simulink model "MotorControlLibSim"  (R2020b)
settings: Solver=FixedStepDiscrete  StartTime=0.0  StopTime=10  FixedStep=1e-6  RelTol=1e-3
undefined symbols (not defined in the file): BrkPoints, d_q_Voltage_Limiter_max, DiscIntNeverNeededParam, Down, dSoll, Ki_dAxis, Ki_qAxis, Kp_dAxis, Kp_qAxis, NumBits1, NumBits2, polepairs, pwmTableData, qSoll, Slope1, Slope2, TqToIqConst, Ts, Up
libraries: simulink x6, eePwmGenerator x3, simulink_extras x2, autolibpmsminterior x1
settings Model: DataDictionary=MotorControl.sldd  NumberOfSteps=10  Creator=unix  LastModifiedBy=unix
settings SolverCC: AutoInsertRateTranBlk=on
settings OptimizationCC: DefaultParameterBehavior=Inlined  EnhancedBackFolding=on  PassReuseOutputArgsAs=Individual arguments  ZeroExternalMemoryAtStartup=off  ZeroInternalMemoryAtStartup=off  OptimizeBlockOrder=speed  DifferentSizesBufferReuse=on  OptimizationCustomize=off  EfficientTunableParamExpr=on
settings DebuggingCC: ArrayBoundsChecking=warning  SignalInfNanChecking=warning  SignalRangeChecking=warning  CheckMatrixSingularityMsg=warning  IntegerOverflowMsg=error  ParameterOverflowMsg=warning  ParameterUnderflowMsg=warning  ParameterPrecisionLossMsg=none  ParameterTunabilityLossMsg=error  UnderSpecifiedDataTypeMsg=warning  IntegerSaturationMsg=error
settings SFSimCC: MATLABDynamicMemAlloc=off
settings RTWCC: Description=Embedded Coder  SystemTargetFile=ert.tlc  GenCodeOnly=on  TemplateMakefile=ert_default_tmf  GenerateReport=on  IncludeHyperlinkInReport=on  LaunchReport=on  GenerateTraceInfo=on  GenerateTraceReport=on  GenerateTraceReportSl=on  GenerateTraceReportSf=on  GenerateTraceReportEml=on
settings CodeAppCC: ForceParamTrailComments=on  IgnoreCustomStorageClasses=off  OperatorAnnotations=on  SimulinkDataObjDesc=on  SFDataObjDesc=on  InsertBlockDesc=on
settings ERTTargetCC: TargetLangStandard=C99 (ISO)  GenerateSampleERTMain=on  GenerateASAP2=on  InlinedParameterPlacement=NonHierarchical  ERTCustomFileTemplate=example_file_process.tlc

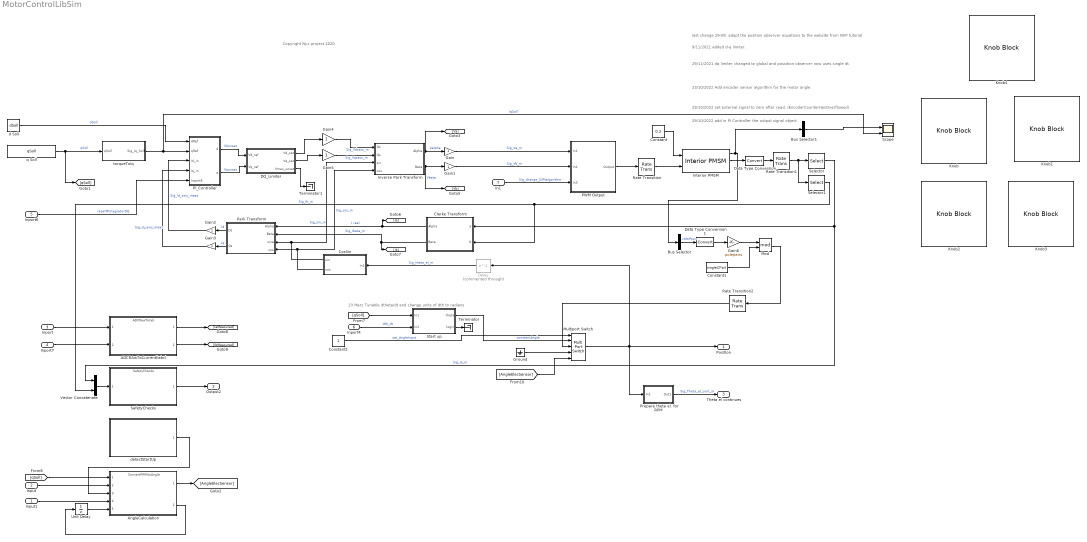
== system MotorControlLibSim ==
  note: Copyright Nyx project 2020
  note: 29/11/2021 dq limiter changed to global and possition observer now uses single dt.
  note: 9/11/2021 added d-q limiter.
  note: last change 29-08: adapt the position observer equations to the website from NXP tutorial
  note: 23 Marz Tunable dtheta/dt and change units of dth to radians
  note: 23/10/2022 Add encoder sensor algorithm for the motor angle
  note: 29/10/2022 set external signal to zero after read, (EncoderCounterHasOverflowed)
  note: 29/10/2022 add in PI Controller the output signal object
  Input1 : Inport
  Input : Inport  Port=2
  Inport : Inport  Port=3
  Inport7 : Inport  Port=4
  Inport6 : Inport  Port=5  OutDataTypeStr=boolean
  Inport4 : Inport  Port=6
  In1 : Inport  Port=7
  ADCRAwToCurrent(Iabc) : ModelReference  ModelNameDialog=ADCRawToIab  ModelReferenceVersion=3.11
  AngleCalculation : ModelReference  ModelNameDialog=ConvertPWMtoAngle.slx  ModelReferenceVersion=3.7
  Bus Selector : BusSelector  OutputSignals=MtrPos
  Bus Selector1 : BusSelector  OutputSignals=MtrPos,IcStator,IbStator,IaStator  OutputAsBus=on
  Clarke Transform : Subsystem  VariantControl=Variant2  mask(Clarke Transform){}
      mask help:
      | <p>Compute Clarke transformation on balanced 3-phase inputs into balanced 2-phase orthogonal outputs.
      | <br>
      | <br>
      | The block accepts two signals out of three phases, and outputs corresponding &alpha;-&beta; axis components, where phase-a axis is aligned with alpha axis.</p>
      mask Help: eval('mcb.internal.helpview(''clarketransform'')')
      mask Display: mcb.internal.drawIcons('Clarke',1);
  Constant : Constant  Value=0.2
  Constant1 : Constant  Value=single(2*pi)  OutDataTypeStr=single
  Constant2 : Constant
  CosSin : Subsystem
  DQ_Limiter : Subsystem  TreatAsAtomicUnit=on  SystemSampleTime=4*Ts  mask(DQ Limiter){Vmax=d_q_Voltage_Limiter_max}
      mask prompts: Vmax "D-Q saturation limit:"
      mask help:
      | Implement saturation on reference dq voltages, with respect to phase voltage peak limit.
      |
      | The block accepts reference values of d and q axis voltages, and outputs corresponding saturated values along with unsaturated peak value to initiate field weakening control.
      |
      | Enter the phase voltage peak limit in the dialog box to initiate saturation.
      settings: RTWFcnNameOpts=Use subsystem name
      mask Help: eval('mcb.internal.helpview(''dqlimiter'')')
  Data Type Conversion : DataTypeConversion
  Data Type Conversion1 : DataTypeConversion
  Delay : Delay  Commented=through  DelayLength=1  SampleTime=4*Ts
      settings: AttributesFormatString=%<SampleTime>
  Gain{,1..3} (4 alike) : Gain  OutDataTypeStr=Inherit: Same as input  ParamDataTypeStr=Inherit: Same as input
  Gain4 : Gain  OutDataTypeStr=Inherit: Inherit via back propagation
  Gain5 : Gain  OutDataTypeStr=Inherit: Inherit via back propagation
  Gain6 : Gain  Gain=polepairs
  Ground : Ground
  Interior PMSM : autolibpmsminterior/Interior PMSM  port_config=Torque  sim_type=Discrete  Ts=1e-6  P=4  Rs=0.0479  Ldq=[8.32e-5 1.07e-4]  KConstText=Back-emf constant (Ke):  lambda_pm=0.2205  Ke=5.2  mechanical=[2.04e-5,4.924e-4,0]  idq0=[0 0]  theta_init=0  omega_init=0  KConst=5.2  lambda_pm_calc=0.0071673  Kt=0.07  RefBlkName='autolibpmsminterior/Interior PMSM'  aMode=5
      settings: SourceProductBaseCode=PW,MT,UV,VE,VP
  Inverse Park Transform : Subsystem  SystemSampleTime=250*Ts  mask(Inverse Park Transform){AxisAlignment=Q-axis}
      mask prompts: AxisAlignment "Alpha (phase-a) axis alignment:"
      mask help:
      | <p>Compute Inverse Park transformation on rotating reference frame inputs into stationary reference frame outputs.
      | <br><br>
      | The block accepts the following:
      | <ul>
      | <li>d-q axis components in rotating reference frame</li>
      | <li>Sine and cosine values of corresponding angle of transformation</li>
      | </ul>
      | The block outputs &alpha;-&beta; axis components in stationary reference frame.
      | <br><br>
      | D-axis alignment with alpha (phase-a) is popular in motor control theory while Q-axis alignment with alpha (phase-a) is more suitable for power conversion applications.</p>
      mask Help: eval('mcb.internal.helpview(''inverseparktransform'')')
      mask TypeOptions AxisAlignment: D-axis | Q-axis
  Knob{,1..4} (5 alike) : KnobBlock  ScaleMax=3
  Mod : Math  Operator=mod  OutputSignalType=real  SaturateOnIntegerOverflow=on
  Multiport Switch : MultiPortSwitch  DataPortOrder=Zero-based contiguous  Inputs=4  zeroidx=on
  PI_Controller : Subsystem  TreatAsAtomicUnit=on  SystemSampleTime=4*Ts
      settings: RTWFcnNameOpts=Use subsystem name
  PWM Output : Subsystem
  Park Transform : Subsystem  SystemSampleTime=250*Ts  mask(Park Transform){AxisAlignment=Q-axis}
      mask prompts: AxisAlignment "Alpha (phase-a) axis alignment:"
      mask help:
      | <p>Compute Park transformation on stationary reference frame inputs into rotating reference frame outputs.
      | <br><br>
      | The block accepts the following:
      | <ul>
      |   <li>&alpha;-&beta; axis components in stationary reference frame</li>
      |   <li>Sine and cosine values of corresponding angle of transformation</li>
      | </ul>
      | The block outputs direct and quadrature axis components in rotating reference frame.
      | <br><br>
      | D-axis alignment with alpha (phase-a) is popular in motor control theory while Q-axis alignment with alpha (phase-a) is more suitable for power conversion applications.</p>
      mask Help: eval('mcb.internal.helpview(''parktransform'')')
      mask TypeOptions AxisAlignment: D-axis | Q-axis
      mask Display: mcb.internal.drawIcons('Park',1);
  Prepare theta el. for RPM : Subsystem
  Rate Transition : RateTransition
  Rate Transition1 : RateTransition
  Rate Transition2 : RateTransition
  SafetyChecks : ModelReference  ModelNameDialog=SafetyChecks.slx  ModelReferenceVersion=1.19
  Scope : Scope  NumInputPorts=2
  Selector : Selector  InputPortWidth=3  IndexOptions=Index vector (dialog)  Indices=1  OutputSizes=1
  Selector1 : Selector  InputPortWidth=3  IndexOptions=Index vector (dialog)  Indices=2  OutputSizes=1
  Start up : Subsystem  TreatAsAtomicUnit=on  SystemSampleTime=4*Ts
  Terminator : Terminator
  Terminator1 : Terminator
  Unit Delay : UnitDelay  SampleTime=-1  HasFrameUpgradeWarning=on
  Vector Concatenate : Concatenate
  d Soll : Constant  Value=dSoll
  detectStartUp : Subsystem  TreatAsAtomicUnit=on  SystemSampleTime=4*Ts  ReferencedSubsystem=detectStartUp
  q Soll : Constant  Value=qSoll
  torqueToIq : Subsystem
  Position : Outport
  Output2 : Outport  Port=2
  Theta el continues : Outport  Port=3
  wires:
  Selector1/1 -> Clarke Transform/2(b), Vector Concatenate/2  "Sig_Ib_m"
  Selector/1 -> Clarke Transform/1(a), Vector Concatenate/1  "Sig_Ia_m"
  Clarke Transform/1(Alpha) -> [Ia], Park Transform/1(Alpha)  "I real"
  Clarke Transform/2(Beta) -> [Ib], Park Transform/2(Beta)  "Sig_Ibeta_m"
  Inverse Park Transform/1(Alpha) -> [Va], Gain/1  "Valpha"
  Gain4/1 -> Inverse Park Transform/1(Ds)  "Sig_Vdsatu_m"
  Gain5/1 -> Inverse Park Transform/2(Qs)  "Sig_Vqsatu_m"
  Inverse Park Transform/2(Beta) -> [Vb], Gain1/1  "Vbeta"
  d Soll/1 -> PI_Controller/1(dRef)  "dSoll"
  PI_Controller/1(d) -> DQ_Limiter/1(Vd_ref)  "Vdunsat"
  PI_Controller/2(q) -> DQ_Limiter/2(Vq_ref)  "Vqunsat"
  Park Transform/2(Qs) -> Gain3/1  "Iq"
  Park Transform/1(Ds) -> Gain2/1  "Id"
  q Soll/1 -> [qSoll], torqueToIq/1(qSoll)  "qSoll"
  ADCRAwToCurrent(Iabc)/2 -> [IbMeasured]
  Inport/1 -> ADCRAwToCurrent(Iabc)/1
  ADCRAwToCurrent(Iabc)/1 -> [IaMeasured]
  CosSin/1(sin) -> Inverse Park Transform/3(sin), Park Transform/3(sine)  "Sig_sin_m"
  CosSin/2(cos) -> Park Transform/4(cos), Inverse Park Transform/4(cos)  "Sig_cos_m"
  Delay/1 -> CosSin/1(In1)  "Sig_theta_el_m"
  Gain/1 -> PWM Output/1(In1)  "Sig_Va_m"
  Gain1/1 -> PWM Output/2(In2)  "Sig_Vb_m"
  Gain2/1 -> PI_Controller/3(Id_in)  "Sig_Id_axis_meas"
  Gain3/1 -> PI_Controller/4(Iq_in)  "Sig_Iq_axis_meas"
  [qSoll] -> Start up/1(In1)
  Start up/1(theta) -> Multiport Switch/2  "constantAngle"
  Start up/2(logic) -> Terminator/1
  Constant2/1 -> Multiport Switch/1  "set_AngleInput"
  Inport4/1 -> Start up/2(In2)  "dth_dt"
  DQ_Limiter/2(Vq_sat) -> Gain5/1
  DQ_Limiter/1(Vd_sat) -> Gain4/1
  DQ_Limiter/3(Vmax_unsat) -> Terminator1/1
  In1/1 -> PWM Output/3(In3)  "Sig_change_SVMalgorithm"
  Multiport Switch/1 -> Delay/1, Position/1, Prepare theta el. for RPM/1(In1)
  Inport6/1 -> PI_Controller/5(Inport6)  "resetPIIntegratorDQ"
  Vector Concatenate/1 -> SafetyChecks/1
  SafetyChecks/1 -> Output2/1
  Inport7/1 -> ADCRAwToCurrent(Iabc)/2
  torqueToIq/1(Sig_Iq_Soll) -> Scope/2, PI_Controller/2(qRef)  "IqSoll"
  Prepare theta el. for RPM/1(Out1) -> Theta el continues/1  "Sig_Theta_el_cont_m"
  Input/1 -> AngleCalculation/2
  detectStartUp/1 -> AngleCalculation/3
  Unit Delay/1 -> AngleCalculation/5
  Input1/1 -> AngleCalculation/4
  [qSoll] -> AngleCalculation/1
  AngleCalculation/2 -> Unit Delay/1
  AngleCalculation/1 -> [AngleElecSensor]
  [AngleElecSensor] -> Multiport Switch/5
  Constant/1 -> Interior PMSM/1
  PWM Output/1(Output) -> Rate Transition/1
  Interior PMSM/2 -> Data Type Conversion/1
  Rate Transition/1 -> Interior PMSM/2
  Rate Transition1/1 -> Selector1/1, Selector/1
  Data Type Conversion/1 -> Rate Transition1/1
  Interior PMSM/1 -> Bus Selector1/1, Bus Selector/1
  Bus Selector/1 -> Data Type Conversion1/1  "<MtrPos>"
  Gain6/1 -> Mod/1
  Constant1/1 -> Mod/2
  Mod/1 -> Rate Transition2/1
  Rate Transition2/1 -> Multiport Switch/3
  Ground/1 -> Multiport Switch/4
  Data Type Conversion1/1 -> Gain6/1
  Bus Selector1/1 -> Scope/1

== system MotorControlLibSim/Clarke Transform ==
  a : Inport
  b : Inport  Port=2
  Data Type Duplicate : DataTypeDuplicate
  a_plus_2b : Sum  Inputs=+++  RndMeth=Simplest  OutDataTypeStr=Inherit: Same as first input
  one_by_sqrt3 : Gain  Gain=1/sqrt(3)  RndMeth=Simplest  OutDataTypeStr=Inherit: Same as input
  Alpha : Outport  VectorParamsAs1DForOutWhenUnconnected=off
  Beta : Outport  Port=2  VectorParamsAs1DForOutWhenUnconnected=off
  wires:
  a/1 -> a_plus_2b/1, Alpha/1, Data Type Duplicate/1
  one_by_sqrt3/1 -> Beta/1
  a_plus_2b/1 -> one_by_sqrt3/1
  b/1 -> a_plus_2b/2, a_plus_2b/3, Data Type Duplicate/2

== system MotorControlLibSim/CosSin ==
  In1 : Inport
  Data Type Conversion1 : DataTypeConversion
  Sine-Cosine Lookup : Subsystem  mask(Sine-Cosine Lookup){AngleInput=Radians, N_points=512}
      mask prompts: AngleInput "Theta units:"; N_points "Number of data points for lookup table:"
      mask help:
      | Implement sine and cosine functions using a lookup table approach for optimized performance on target hardware.
      |
      | The block accepts input angle in different units and outputs corresponding sine and cosine values.
      mask init:
      | % dlgSett = mct.internal.SinCosCb(gcbh);
      | this = get_param(gcbh,'Object');
      | 
      | points = eval(this.N_points);
      | 
      | dlgSett.points = 125*floor(points/125);
      | 
      | dlgSett.Offset = uint16(dlgSett.points/5);
      | 
      | dlgSett.N_points = 4*dlgSett.Offset;
      | N_points = dlgSett.N_points;
      | 
      | theta = linspace(0,2*pi,N_points+1);
      | dlgSett.size = 5*dlgSett.Offset+2;
      | dlgSett.sin_table = zeros(1,dlgSett.size);
      | dlgSett.sin_table(1:N_points+1) = sin(theta);
      | dlgSett.sin_table(N_points+2:dlgSett.size) = dlgSett.sin_table(2:0.25*N_points+2);
      | 
      | dlgSett.N_points = double(dlgSett.N_points);
      | dlgSett.index_gain = dlgSett.N_points;
      | dlgSett.UpperSatLimit = 1;
      | 
      | switch AngleInput
      |     case 1
      |         dlgSett.UpperSatLimit = 1;
      |     case 2
      |         dlgSett.UpperSatLimit = 2*pi;
      |     case 3
      |         dlgSett.UpperSatLimit = 360;
      |     otherwise
      | end
      mask Help: eval('mcb.internal.helpview(''sinecosinelookup'')')
      mask TypeOptions AngleInput: Per-unit | Radians | Degrees
      mask Display: mcb.internal.drawIcons('Sin-Cos',1);
  sin : Outport
  cos : Outport  Port=2
  wires:
  Sine-Cosine Lookup/2(cos) -> cos/1
  In1/1 -> Data Type Conversion1/1
  Sine-Cosine Lookup/1(sin) -> sin/1
  Data Type Conversion1/1 -> Sine-Cosine Lookup/1(Theta)

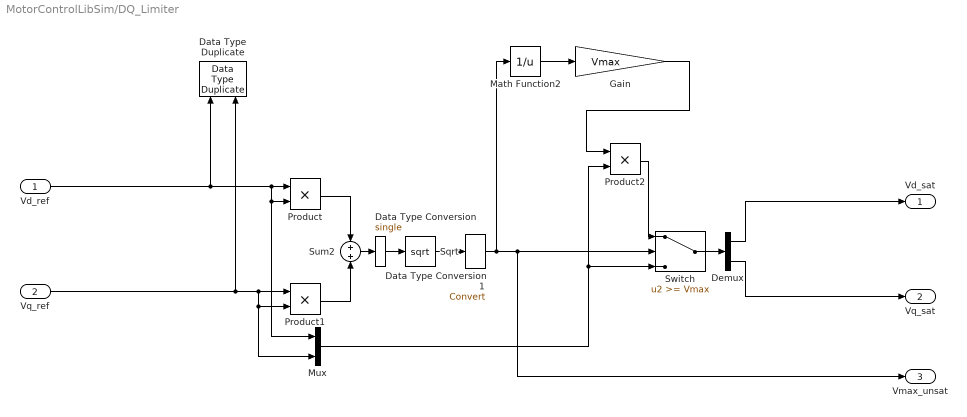
== system MotorControlLibSim/DQ_Limiter ==
  Vd_ref : Inport
  Vq_ref : Inport  Port=2
  Data Type Duplicate : DataTypeDuplicate
  Data Type Conversion : DataTypeConversion  OutDataTypeStr=single
  Data Type Conversion1 : DataTypeConversion
  Demux : Demux  Outputs=2
  Gain : Gain  Gain=Vmax  OutDataTypeStr=Inherit: Same as input
  Math Function2 : Math  Operator=reciprocal  SignedPower=on  RndMeth=Simplest
  Mux : Mux  Inputs=2
  Product : Product  RndMeth=Simplest  OutDataTypeStr=Inherit: Same as first input
  Product1 : Product  RndMeth=Simplest  OutDataTypeStr=Inherit: Same as first input
  Product2 : Product  OutDataTypeStr=Inherit: Same as first input
  Sqrt : Sqrt  IntermediateResultsDataTypeStr=Inherit: Inherit from input  SaturateOnIntegerOverflow=on
  Sum2 : Sum  OutDataTypeStr=Inherit: Same as first input
  Switch : Switch  Threshold=Vmax  ZeroCross=off
  Vd_sat : Outport  VectorParamsAs1DForOutWhenUnconnected=off
  Vq_sat : Outport  Port=2  VectorParamsAs1DForOutWhenUnconnected=off
  Vmax_unsat : Outport  Port=3  VectorParamsAs1DForOutWhenUnconnected=off
  wires:
  Vd_ref/1 -> Data Type Duplicate/1, Product/1, Product/2, Mux/1
  Demux/1 -> Vd_sat/1
  Product1/1 -> Sum2/2
  Product/1 -> Sum2/1
  Sum2/1 -> Data Type Conversion/1
  Math Function2/1 -> Gain/1
  Mux/1 -> Product2/2, Switch/3
  Product2/1 -> Switch/1
  Switch/1 -> Demux/1
  Demux/2 -> Vq_sat/1
  Sqrt/1 -> Data Type Conversion1/1
  Gain/1 -> Product2/1
  Vq_ref/1 -> Data Type Duplicate/2, Product1/1, Product1/2, Mux/2
  Data Type Conversion1/1 -> Vmax_unsat/1, Switch/2, Math Function2/1
  Data Type Conversion/1 -> Sqrt/1

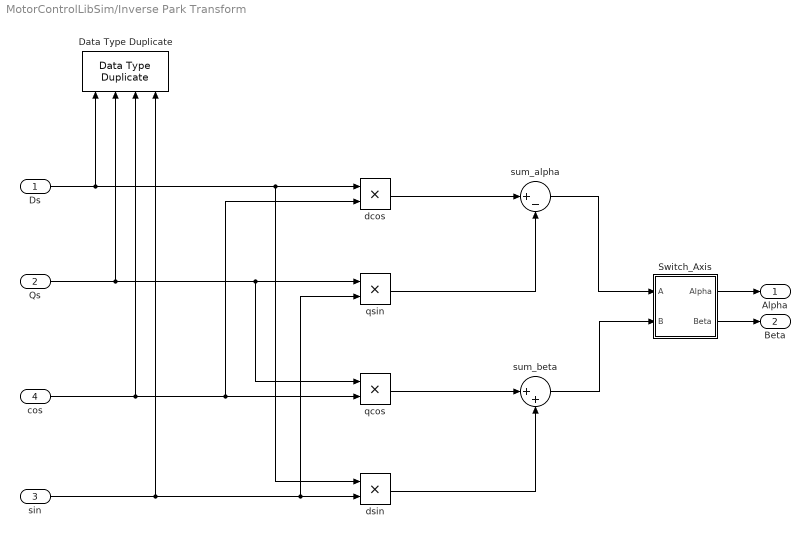
== system MotorControlLibSim/Inverse Park Transform ==
  Ds : Inport
  Qs : Inport  Port=2
  sin : Inport  Port=3
  cos : Inport  Port=4
  Data Type Duplicate : DataTypeDuplicate  NumInputPorts=4
  Switch_Axis : Subsystem
  dcos : Product  RndMeth=Simplest  OutDataTypeStr=Inherit: Same as first input
  dsin : Product  RndMeth=Simplest  OutDataTypeStr=Inherit: Same as first input
  qcos : Product  RndMeth=Simplest  OutDataTypeStr=Inherit: Same as first input
  qsin : Product  RndMeth=Simplest  OutDataTypeStr=Inherit: Same as first input
  sum_alpha : Sum  Inputs=|+-  RndMeth=Simplest  OutDataTypeStr=Inherit: Same as first input
  sum_beta : Sum  Inputs=|++  RndMeth=Simplest  OutDataTypeStr=Inherit: Same as first input
  Alpha : Outport  VectorParamsAs1DForOutWhenUnconnected=off
  Beta : Outport  Port=2  VectorParamsAs1DForOutWhenUnconnected=off
  wires:
  Switch_Axis/2(Beta) -> Beta/1
  Switch_Axis/1(Alpha) -> Alpha/1
  sum_beta/1 -> Switch_Axis/2(B)
  sum_alpha/1 -> Switch_Axis/1(A)
  sin/1 -> dsin/2, qsin/2, Data Type Duplicate/4
  cos/1 -> qcos/2, dcos/2, Data Type Duplicate/3
  dsin/1 -> sum_beta/2
  Qs/1 -> qsin/1, qcos/1, Data Type Duplicate/2
  dcos/1 -> sum_alpha/1
  qcos/1 -> sum_beta/1
  qsin/1 -> sum_alpha/2
  Ds/1 -> dcos/1, dsin/1, Data Type Duplicate/1

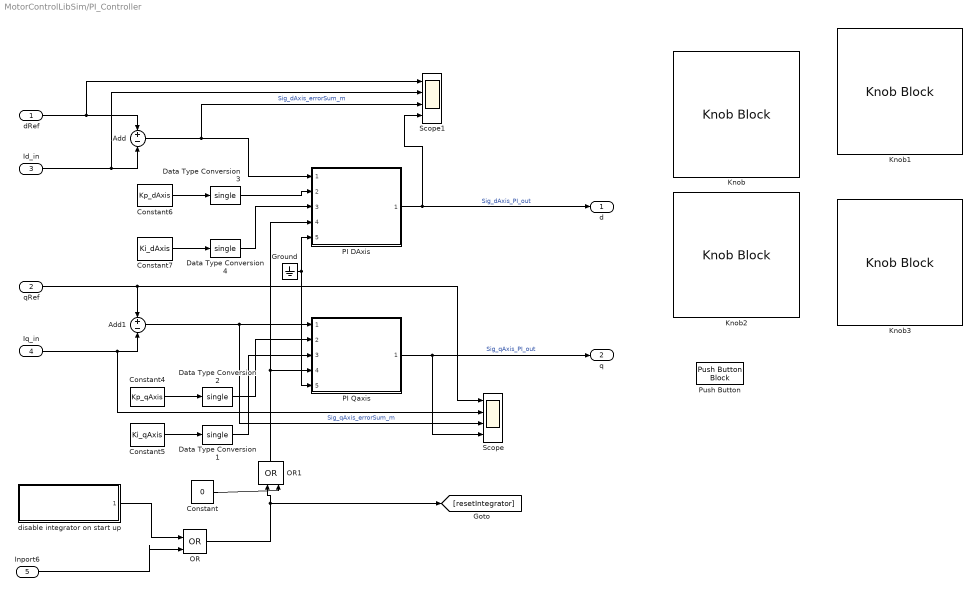
== system MotorControlLibSim/PI_Controller ==
  dRef : Inport
  qRef : Inport  Port=2
  Id_in : Inport  Port=3
  Iq_in : Inport  Port=4
  Inport6 : Inport  Port=5
  Add : Sum  Inputs=+|-  RndMeth=Simplest
  Add1 : Sum  Inputs=+|-  RndMeth=Simplest
  Constant : Constant  Value=0  OutDataTypeStr=boolean
  Constant4 : Constant  Value=Kp_qAxis
  Constant5 : Constant  Value=Ki_qAxis
  Constant6 : Constant  Value=Kp_dAxis
  Constant7 : Constant  Value=Ki_dAxis
  Data Type Conversion{1..4} (4 alike) : DataTypeConversion  OutDataTypeStr=single
  Ground : Ground
  Knob : KnobBlock  ScaleMax=1
  Knob1 : KnobBlock  ScaleMax=1
  Knob2 : KnobBlock  ScaleMax=200
  Knob3 : KnobBlock  ScaleMax=200
  OR : Logic  Operator=OR  IconShape=distinctive  AllPortsSameDT=off  OutDataTypeStr=boolean
  OR1 : Logic  Operator=OR  IconShape=distinctive  AllPortsSameDT=off  OutDataTypeStr=boolean
  PI DAxis : Subsystem  TreatAsAtomicUnit=on  ReferencedSubsystem=PID_custom
  PI Qaxis : Subsystem  TreatAsAtomicUnit=on  ReferencedSubsystem=PID_custom
  Push Button : PushButtonBlock
  Scope : Scope  NumInputPorts=4
  Scope1 : Scope  NumInputPorts=4
  disable integrator on start up : Subsystem  ReferencedSubsystem=disable_integrator_on_start_up
  d : Outport
  q : Outport  Port=2
  wires:
  qRef/1 -> Scope/1, Add1/1
  Iq_in/1 -> Scope/2, Add1/2
  PI Qaxis/1 -> Scope/4, q/1  "Sig_qAxis_PI_out"
  Id_in/1 -> Scope1/2, Add/2
  Add1/1 -> Scope/3, PI Qaxis/1  "Sig_qAxis_errorSum_m"
  Constant5/1 -> Data Type Conversion1/1
  Constant4/1 -> Data Type Conversion2/1
  disable integrator on start up/1 -> OR/1
  Inport6/1 -> OR/2
  Data Type Conversion1/1 -> PI Qaxis/3
  Data Type Conversion2/1 -> PI Qaxis/2
  Add/1 -> Scope1/3, PI DAxis/1  "Sig_dAxis_errorSum_m"
  Constant6/1 -> Data Type Conversion3/1
  Constant7/1 -> Data Type Conversion4/1
  PI DAxis/1 -> Scope1/4, d/1  "Sig_dAxis_PI_out"
  OR/1 -> [resetIntegrator], OR1/1
  Data Type Conversion3/1 -> PI DAxis/2
  Data Type Conversion4/1 -> PI DAxis/3
  dRef/1 -> Scope1/1, Add/1
  Ground/1 -> PI Qaxis/5, PI DAxis/5
  OR1/1 -> PI DAxis/4, PI Qaxis/4
  Constant/1 -> OR1/2

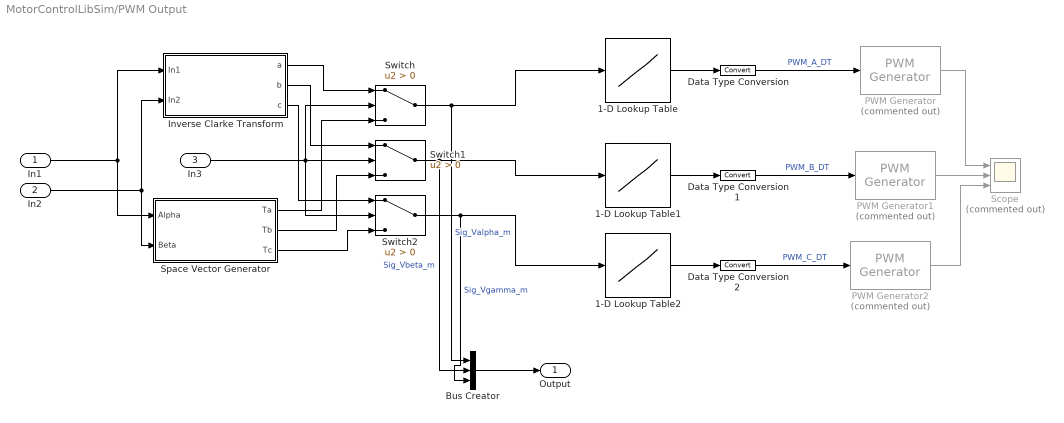
== system MotorControlLibSim/PWM Output ==
  In1 : Inport
  In2 : Inport  Port=2
  In3 : Inport  Port=3
  1-D Lookup Table : Lookup_n-D  NumberOfTableDimensions=1  BreakpointsForDimension1=BrkPoints  Table=pwmTableData  ExtrapMethod=Clip  InternalRulePriority=Speed  OutDataTypeStr=uint16  RndMeth=Simplest  SaturateOnIntegerOverflow=on  InputSameDT=on
  1-D Lookup Table1 : Lookup_n-D  NumberOfTableDimensions=1  BreakpointsForDimension1=BrkPoints  Table=pwmTableData  ExtrapMethod=Clip  InternalRulePriority=Speed  OutDataTypeStr=uint16  RndMeth=Simplest  SaturateOnIntegerOverflow=on  InputSameDT=on
  1-D Lookup Table2 : Lookup_n-D  NumberOfTableDimensions=1  BreakpointsForDimension1=BrkPoints  Table=pwmTableData  ExtrapMethod=Clip  InternalRulePriority=Speed  OutDataTypeStr=uint16  RndMeth=Simplest  SaturateOnIntegerOverflow=on  InputSameDT=on
  Bus Creator : BusCreator  Inputs=3
  Data Type Conversion : DataTypeConversion
  Data Type Conversion1 : DataTypeConversion
  Data Type Conversion2 : DataTypeConversion
  Inverse Clarke Transform : Subsystem  TreatAsAtomicUnit=on  mask(Inverse Clarke Transform){}
      mask help:
      | <p>Compute Inverse Clarke transformation on balanced 2-phase orthogonal inputs into balanced 3-phase outputs.
      | <br><br>
      | The block accepts &alpha;-&beta; axis components and outputs corresponding 3-phase outputs, where phase-a axis is aligned with &alpha;-axis.</p>
      mask Help: eval('mcb.internal.helpview(''inverseclarketransform'')')
      mask Display: mcb.internal.drawIcons('invClarke',1);
  PWM Generator : eePwmGenerator/PWM Generator  Commented=on  CarrCount=Up-Down  Tper=10*Ts  Ts=Ts
  PWM Generator1 : eePwmGenerator/PWM Generator  Commented=on  CarrCount=Up-Down  Tper=10*Ts  Ts=Ts
  PWM Generator2 : eePwmGenerator/PWM Generator  Commented=on  CarrCount=Up-Down  Tper=10*Ts  Ts=Ts
  Scope : Scope  Commented=on  NumInputPorts=3
  Space Vector Generator : Subsystem  TreatAsAtomicUnit=on  mask(Space Vector Generator){}
      mask help:
      | <p>Generate space vector modulation signals from stator reference voltages described by  &alpha;-&beta; components.
      | <br><br>
      | The block accepts V<sub>&alpha;</sub> and V<sub>&beta;</sub> voltages and outputs corresponding space vector modulation voltages.</p>
      mask Help: eval('mcb.internal.helpview(''spacevectorgenerator'')')
      mask Display: mcb.internal.drawIcons('SVPWM',1);
  Switch : Switch  Criteria=u2 > Threshold
  Switch1 : Switch  Criteria=u2 > Threshold
  Switch2 : Switch  Criteria=u2 > Threshold
  Output : Outport
  wires:
  In2/1 -> Space Vector Generator/2(Beta), Inverse Clarke Transform/2(In2)
  In1/1 -> Space Vector Generator/1(Alpha), Inverse Clarke Transform/1(In1)
  Switch/1 -> Bus Creator/1, 1-D Lookup Table/1  "Sig_Valpha_m"
  1-D Lookup Table/1 -> Data Type Conversion/1
  Switch1/1 -> Bus Creator/2, 1-D Lookup Table1/1  "Sig_Vbeta_m"
  Switch2/1 -> Bus Creator/3, 1-D Lookup Table2/1  "Sig_Vgamma_m"
  PWM Generator/1 -> Scope/1
  1-D Lookup Table2/1 -> Data Type Conversion2/1
  1-D Lookup Table1/1 -> Data Type Conversion1/1
  PWM Generator1/1 -> Scope/2
  PWM Generator2/1 -> Scope/3
  Data Type Conversion/1 -> PWM Generator/1  "PWM_A_DT"
  Data Type Conversion1/1 -> PWM Generator1/1  "PWM_B_DT"
  Data Type Conversion2/1 -> PWM Generator2/1  "PWM_C_DT"
  Space Vector Generator/1(Ta) -> Switch/3
  Space Vector Generator/2(Tb) -> Switch1/3
  Space Vector Generator/3(Tc) -> Switch2/3
  Inverse Clarke Transform/1(a) -> Switch/1
  Inverse Clarke Transform/2(b) -> Switch1/1
  Inverse Clarke Transform/3(c) -> Switch2/1
  In3/1 -> Switch/2, Switch2/2, Switch1/2
  Bus Creator/1 -> Output/1

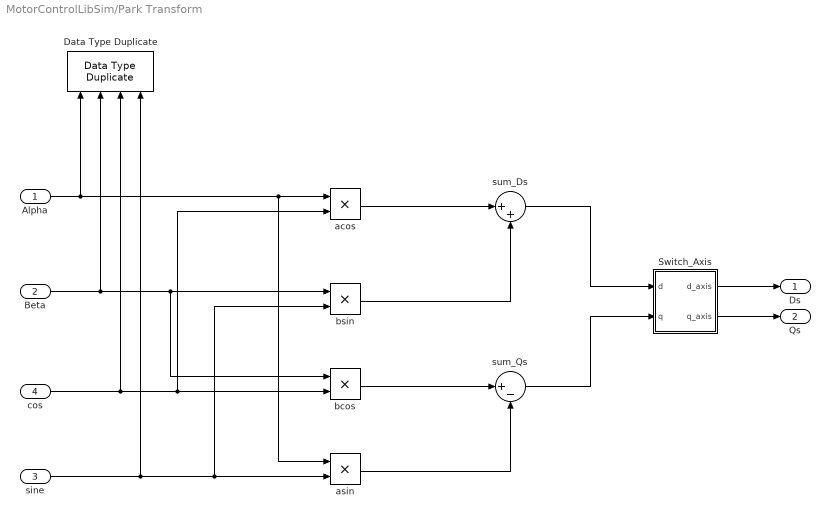
== system MotorControlLibSim/Park Transform ==
  Alpha : Inport
  Beta : Inport  Port=2
  sine : Inport  Port=3
  cos : Inport  Port=4
  Data Type Duplicate : DataTypeDuplicate  NumInputPorts=4
  Switch_Axis : Subsystem
  acos : Product  RndMeth=Simplest  OutDataTypeStr=Inherit: Same as first input
  asin : Product  RndMeth=Simplest  OutDataTypeStr=Inherit: Same as first input
  bcos : Product  OutDataTypeStr=Inherit: Inherit via back propagation  RndMeth=Simplest
  bsin : Product  OutDataTypeStr=Inherit: Inherit via back propagation  RndMeth=Simplest
  sum_Ds : Sum  Inputs=|++  RndMeth=Simplest  OutDataTypeStr=Inherit: Same as first input
  sum_Qs : Sum  Inputs=|+-  RndMeth=Simplest  OutDataTypeStr=Inherit: Same as first input
  Ds : Outport  VectorParamsAs1DForOutWhenUnconnected=off
  Qs : Outport  Port=2  VectorParamsAs1DForOutWhenUnconnected=off
  wires:
  Beta/1 -> Data Type Duplicate/2, bcos/1, bsin/1
  Switch_Axis/1(d_axis) -> Ds/1
  Switch_Axis/2(q_axis) -> Qs/1
  sum_Ds/1 -> Switch_Axis/1(d)
  sum_Qs/1 -> Switch_Axis/2(q)
  cos/1 -> Data Type Duplicate/3, bcos/2, acos/2
  asin/1 -> sum_Qs/2
  bcos/1 -> sum_Qs/1
  bsin/1 -> sum_Ds/2
  acos/1 -> sum_Ds/1
  Alpha/1 -> Data Type Duplicate/1, acos/1, asin/1
  sine/1 -> bsin/2, asin/2, Data Type Duplicate/4

== system MotorControlLibSim/Prepare theta el. for RPM ==
  In1 : Inport
  Add : Sum
  Compare To Constant : simulink/Logic and Bit Operations/Compare To Constant  relop=>  const=400000.0  OutDataTypeStr=boolean
  Constant : Constant  Value=0  OutDataTypeStr=single
  Data Type Conversion : DataTypeConversion  OutDataTypeStr=single
  Switch : Switch  Threshold=1  OutDataTypeStr=single
  Unit Delay : UnitDelay  SampleTime=-1  HasFrameUpgradeWarning=on
  Out1 : Outport
  wires:
  Unit Delay/1 -> Add/2
  Switch/1 -> Unit Delay/1, Data Type Conversion/1
  In1/1 -> Add/1
  Data Type Conversion/1 -> Out1/1
  Add/1 -> Switch/3, Compare To Constant/1
  Compare To Constant/1 -> Switch/2
  Constant/1 -> Switch/1

== system MotorControlLibSim/Start up ==
  In1 : Inport
  In2 : Inport  Port=2
  Logic after motor is stoped : Subsystem
  Simulate start up Theta : Subsystem
  theta : Outport
  logic : Outport  Port=2
  wires:
  In1/1 -> Logic after motor is stoped/1(In1)
  Logic after motor is stoped/1(Out1) -> logic/1
  In2/1 -> Simulate start up Theta/1(In1)
  Simulate start up Theta/1(Out1) -> theta/1

== system MotorControlLibSim/torqueToIq ==
  qSoll : Inport
  Tq--> iqRef : Gain  Gain=TqToIqConst  ParamDataTypeStr=Inherit: Inherit from 'Gain'  OutDataTypeStr=single
  Sig_Iq_Soll : Outport
  wires:
  Tq--> iqRef/1 -> Sig_Iq_Soll/1  "Sig_Iq_Soll"
  qSoll/1 -> Tq--> iqRef/1

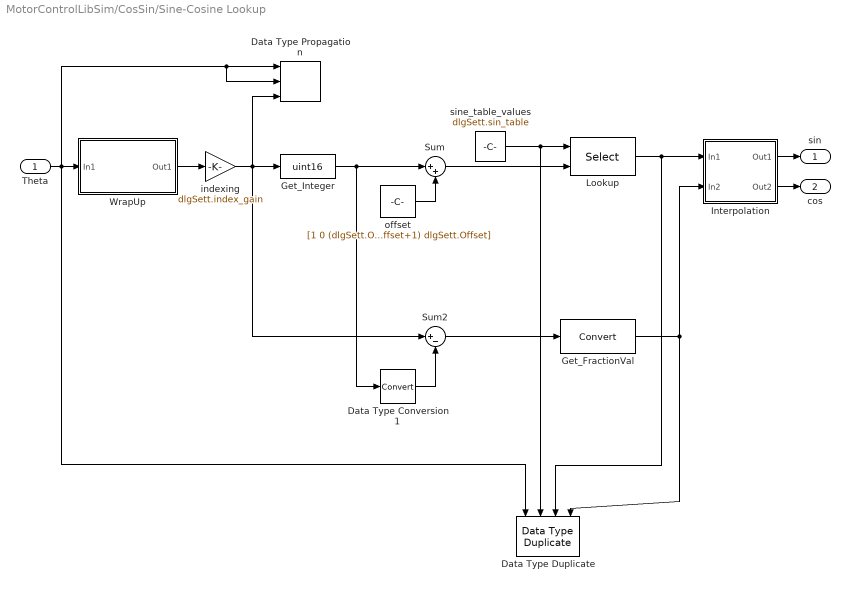
== system MotorControlLibSim/CosSin/Sine-Cosine Lookup ==
  Theta : Inport
  Data Type Duplicate : DataTypeDuplicate  NumInputPorts=4
  Data Type Propagation : simulink/Signal Attributes/Data Type Propagation  PropDataType=fixdt(1, 16)  IfRefDouble=double  IfRefSingle=single  IsSigned=IsSigned1 or IsSigned2  NumBitsBase=max([NumBits1 NumBits2])  NumBitsMult=1  NumBitsAdd=0  NumBitsAllowFinal=1:128  PropScalingMode=Obtain via best precision  PropScaling=2^-10  ValuesUsedBestPrec=[0 dlgSett.index_gain]  SlopeBase=min([Slope1 Slope2])  SlopeMult=1  SlopeAdd=0  BiasBase=Bias1  BiasMult=1  BiasAdd=0
      settings: SourceProductBaseCode=SL
  Data Type Conversion1 : DataTypeConversion  RndMeth=Simplest
  Get_FractionVal : DataTypeConversion  RndMeth=Simplest
  Get_Integer : DataTypeConversion  OutDataTypeStr=uint16  RndMeth=Simplest
  Interpolation : Subsystem
  Lookup : Selector  IndexMode=Zero-based  InputPortWidth=dlgSett.size  IndexOptions=Index vector (port)  Indices=[1 3]  OutputSizes=1
  Sum : Sum  Inputs=|++  AccumDataTypeStr=uint32  OutDataTypeStr=uint32  RndMeth=Simplest
  Sum2 : Sum  Inputs=|+-  RndMeth=Simplest  OutDataTypeStr=Inherit: Same as first input
  WrapUp : Subsystem
  indexing : Gain  Gain=dlgSett.index_gain  OutDataTypeStr=Inherit: Inherit via back propagation  RndMeth=Simplest
  offset : Constant  Value=[1 0 (dlgSett.Offset+1) dlgSett.Offset]  OutDataTypeStr=int16  SampleTime=-1
  sine_table_values : Constant  Value=dlgSett.sin_table  OutDataTypeStr=Inherit: Inherit via back propagation  SampleTime=-1
  sin : Outport  VectorParamsAs1DForOutWhenUnconnected=off
  cos : Outport  Port=2  VectorParamsAs1DForOutWhenUnconnected=off
  wires:
  Interpolation/2(Out2) -> cos/1
  Interpolation/1(Out1) -> sin/1
  Sum/1 -> Lookup/2
  indexing/1 -> Sum2/1, Data Type Propagation/3, Get_Integer/1
  Data Type Conversion1/1 -> Sum2/2
  Get_Integer/1 -> Sum/1, Data Type Conversion1/1
  offset/1 -> Sum/2
  sine_table_values/1 -> Lookup/1, Data Type Duplicate/2
  Lookup/1 -> Interpolation/1(In1), Data Type Duplicate/3
  Sum2/1 -> Get_FractionVal/1
  Get_FractionVal/1 -> Data Type Duplicate/4, Interpolation/2(In2)
  Theta/1 -> Data Type Duplicate/1, WrapUp/1(In1), Data Type Propagation/2, Data Type Propagation/1
  WrapUp/1(Out1) -> indexing/1

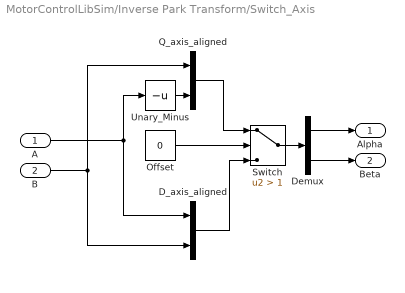
== system MotorControlLibSim/Inverse Park Transform/Switch_Axis ==
  A : Inport
  B : Inport  Port=2
  D_axis_aligned : Mux  Inputs=2
  Demux : Demux  Outputs=2
  Offset : Constant  Value=0  OutDataTypeStr=uint16  SampleTime=-1
  Q_axis_aligned : Mux  Inputs=2
  Switch : Switch  Criteria=u2 > Threshold  Threshold=1  RndMeth=Simplest  ZeroCross=off
  Unary_Minus : UnaryMinus
  Alpha : Outport  VectorParamsAs1DForOutWhenUnconnected=off
  Beta : Outport  Port=2  VectorParamsAs1DForOutWhenUnconnected=off
  wires:
  A/1 -> D_axis_aligned/1, Unary_Minus/1
  Unary_Minus/1 -> Q_axis_aligned/2
  Demux/2 -> Beta/1
  Switch/1 -> Demux/1
  B/1 -> D_axis_aligned/2, Q_axis_aligned/1
  Demux/1 -> Alpha/1
  Offset/1 -> Switch/2
  Q_axis_aligned/1 -> Switch/1
  D_axis_aligned/1 -> Switch/3

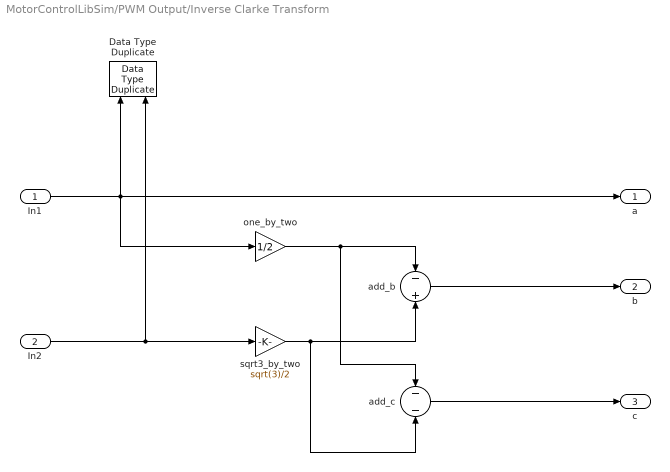
== system MotorControlLibSim/PWM Output/Inverse Clarke Transform ==
  In1 : Inport
  In2 : Inport  Port=2
  Data Type Duplicate : DataTypeDuplicate
  add_b : Sum  Inputs=-+  RndMeth=Simplest  OutDataTypeStr=Inherit: Same as first input
  add_c : Sum  Inputs=--  RndMeth=Simplest  OutDataTypeStr=Inherit: Same as first input
  one_by_two : Gain  Gain=1/2  RndMeth=Simplest  OutDataTypeStr=Inherit: Same as input
  sqrt3_by_two : Gain  Gain=sqrt(3)/2  RndMeth=Simplest  OutDataTypeStr=Inherit: Same as input
  a : Outport  VectorParamsAs1DForOutWhenUnconnected=off
  b : Outport  Port=2  VectorParamsAs1DForOutWhenUnconnected=off
  c : Outport  Port=3  VectorParamsAs1DForOutWhenUnconnected=off
  wires:
  add_c/1 -> c/1
  sqrt3_by_two/1 -> add_c/2, add_b/2
  In1/1 -> one_by_two/1, Data Type Duplicate/1, a/1
  one_by_two/1 -> add_b/1, add_c/1
  In2/1 -> sqrt3_by_two/1, Data Type Duplicate/2
  add_b/1 -> b/1

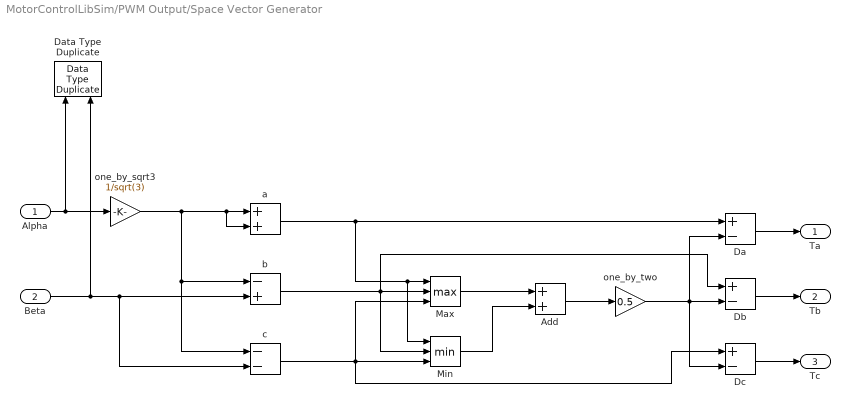
== system MotorControlLibSim/PWM Output/Space Vector Generator ==
  Alpha : Inport
  Beta : Inport  Port=2
  Add : Sum  RndMeth=Simplest  OutDataTypeStr=Inherit: Same as first input
  Da : Sum  Inputs=+-  RndMeth=Simplest  OutDataTypeStr=Inherit: Same as first input
  Data Type Duplicate : DataTypeDuplicate
  Db : Sum  Inputs=+-  RndMeth=Simplest  OutDataTypeStr=Inherit: Same as first input
  Dc : Sum  Inputs=+-  RndMeth=Simplest  OutDataTypeStr=Inherit: Same as first input
  Max : MinMax  Function=max  Inputs=3  RndMeth=Simplest
  Min : MinMax  Inputs=3  RndMeth=Simplest
  a : Sum  RndMeth=Simplest  OutDataTypeStr=Inherit: Same as first input
  b : Sum  Inputs=-+  RndMeth=Simplest  OutDataTypeStr=Inherit: Same as first input
  c : Sum  Inputs=--  RndMeth=Simplest  OutDataTypeStr=Inherit: Same as first input
  one_by_sqrt3 : Gain  Gain=1/sqrt(3)  RndMeth=Simplest  OutDataTypeStr=Inherit: Same as input  ParamDataTypeStr=Inherit: Same as input
  one_by_two : Gain  Gain=0.5  RndMeth=Simplest  OutDataTypeStr=Inherit: Same as input  ParamDataTypeStr=Inherit: Same as input
  Ta : Outport  VectorParamsAs1DForOutWhenUnconnected=off
  Tb : Outport  Port=2  VectorParamsAs1DForOutWhenUnconnected=off
  Tc : Outport  Port=3  VectorParamsAs1DForOutWhenUnconnected=off
  wires:
  Db/1 -> Tb/1
  Dc/1 -> Tc/1
  Da/1 -> Ta/1
  a/1 -> Max/1, Min/1, Da/1
  Max/1 -> Add/1
  one_by_two/1 -> Da/2, Db/2, Dc/2
  Add/1 -> one_by_two/1
  Min/1 -> Add/2
  Alpha/1 -> Data Type Duplicate/1, one_by_sqrt3/1
  one_by_sqrt3/1 -> a/1, a/2, b/1, c/1
  Beta/1 -> c/2, b/2, Data Type Duplicate/2
  b/1 -> Max/2, Min/2, Db/1
  c/1 -> Min/3, Dc/1, Max/3

== system MotorControlLibSim/Park Transform/Switch_Axis ==
  d : Inport
  q : Inport  Port=2
  D_axis_aligned : Mux  Inputs=2
  Demux : Demux  Outputs=2
  Offset : Constant  Value=0  OutDataTypeStr=uint16  SampleTime=-1
  Q_axis_aligned : Mux  Inputs=2
  Switch : Switch  Criteria=u2 > Threshold  Threshold=1  RndMeth=Simplest  ZeroCross=off
  Unary_Minus : UnaryMinus
  d_axis : Outport  VectorParamsAs1DForOutWhenUnconnected=off
  q_axis : Outport  Port=2  VectorParamsAs1DForOutWhenUnconnected=off
  wires:
  D_axis_aligned/1 -> Switch/3
  Q_axis_aligned/1 -> Switch/1
  d/1 -> D_axis_aligned/1, Q_axis_aligned/2
  Offset/1 -> Switch/2
  Demux/1 -> d_axis/1
  Unary_Minus/1 -> Q_axis_aligned/1
  q/1 -> D_axis_aligned/2, Unary_Minus/1
  Switch/1 -> Demux/1
  Demux/2 -> q_axis/1

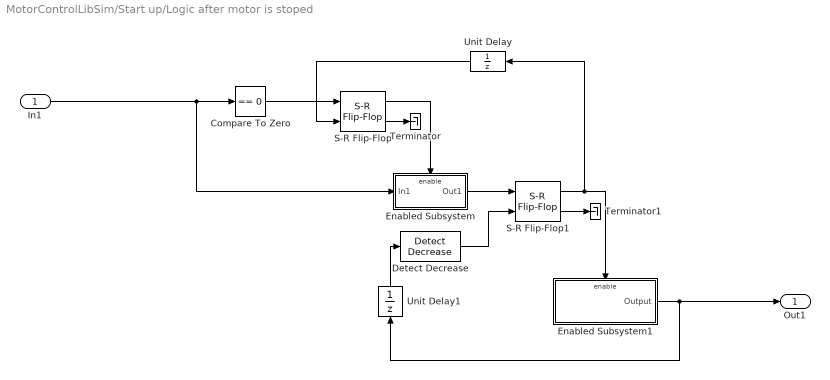
== system MotorControlLibSim/Start up/Logic after motor is stoped ==
  In1 : Inport
  Compare To Zero : simulink/Logic and Bit Operations/Compare To Zero  relop===  OutDataTypeStr=boolean
  Detect Decrease : simulink/Logic and Bit Operations/Detect Decrease  vinit=0  OutDataTypeStr=boolean
  Enabled Subsystem : Subsystem  TreatAsAtomicUnit=on
  Enabled Subsystem1 : Subsystem  TreatAsAtomicUnit=on
  S-R Flip-Flop : simulink_extras/Flip Flops/S-R Flip-Flop  initial_condition=0
  S-R Flip-Flop1 : simulink_extras/Flip Flops/S-R Flip-Flop  initial_condition=0
  Terminator : Terminator
  Terminator1 : Terminator
  Unit Delay : UnitDelay  SampleTime=-1  HasFrameUpgradeWarning=on
  Unit Delay1 : UnitDelay  SampleTime=-1  HasFrameUpgradeWarning=on
  Out1 : Outport
  wires:
  Enabled Subsystem/1(Out1) -> S-R Flip-Flop1/1
  In1/1 -> Enabled Subsystem/1(In1), Compare To Zero/1
  S-R Flip-Flop/2 -> Terminator/1
  Enabled Subsystem1/1(Output) -> Out1/1, Unit Delay1/1
  S-R Flip-Flop/1 -> Enabled Subsystem/Enable
  S-R Flip-Flop1/1 -> Enabled Subsystem1/Enable, Unit Delay/1
  Unit Delay/1 -> S-R Flip-Flop/2
  Compare To Zero/1 -> S-R Flip-Flop/1
  S-R Flip-Flop1/2 -> Terminator1/1
  Unit Delay1/1 -> Detect Decrease/1
  Detect Decrease/1 -> S-R Flip-Flop1/2

== system MotorControlLibSim/Start up/Simulate start up Theta ==
  note: Overflow danger
  In1 : Inport
  Abs : Abs
  Constant : Constant  Value=2*pi  OutDataTypeStr=fixdt(1,16,2^-8,0)
  Discrete-Time Integrator : DiscreteIntegrator  ExternalReset=rising  SampleTime=-1  OutDataTypeStr=fixdt(1,16,2^-8,0)  ICPrevOutput=DiscIntNeverNeededParam  ICPrevScaledInput=DiscIntNeverNeededParam
  Relational Operator : RelationalOperator  OutDataTypeStr=boolean  RndMeth=Simplest
  Unit Delay : UnitDelay  SampleTime=-1  HasFrameUpgradeWarning=on
  Out1 : Outport
  wires:
  Constant/1 -> Relational Operator/2
  Relational Operator/1 -> Unit Delay/1
  Unit Delay/1 -> Discrete-Time Integrator/2
  In1/1 -> Discrete-Time Integrator/1
  Discrete-Time Integrator/1 -> Out1/1, Abs/1
  Abs/1 -> Relational Operator/1

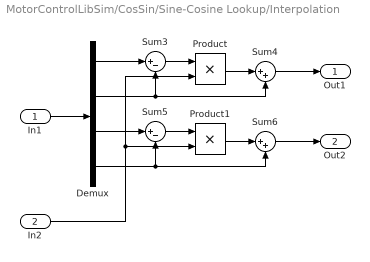
== system MotorControlLibSim/CosSin/Sine-Cosine Lookup/Interpolation ==
  In1 : Inport
  In2 : Inport  Port=2
  Demux : Demux
  Product : Product  RndMeth=Simplest  OutDataTypeStr=Inherit: Same as first input
  Product1 : Product  RndMeth=Simplest  OutDataTypeStr=Inherit: Same as first input
  Sum3 : Sum  Inputs=|+-  RndMeth=Simplest  OutDataTypeStr=Inherit: Same as first input
  Sum4 : Sum  Inputs=|++  RndMeth=Simplest  OutDataTypeStr=Inherit: Same as first input
  Sum5 : Sum  Inputs=|+-  RndMeth=Simplest  OutDataTypeStr=Inherit: Same as first input
  Sum6 : Sum  Inputs=|++  RndMeth=Simplest  OutDataTypeStr=Inherit: Same as first input
  Out1 : Outport
  Out2 : Outport  Port=2
  wires:
  Sum4/1 -> Out1/1
  Sum6/1 -> Out2/1
  Demux/1 -> Sum3/1
  Sum5/1 -> Product1/1
  Demux/2 -> Sum3/2, Sum4/2
  In2/1 -> Product/2, Product1/2
  Product/1 -> Sum4/1
  Demux/4 -> Sum6/2, Sum5/2
  Product1/1 -> Sum6/1
  In1/1 -> Demux/1
  Sum3/1 -> Product/1
  Demux/3 -> Sum5/1

== system MotorControlLibSim/CosSin/Sine-Cosine Lookup/WrapUp ==
  In1 : Inport
  Compare To Zero : simulink/Logic and Bit Operations/Compare To Zero  relop=<  OutDataTypeStr=boolean
  Data Type Conversion : DataTypeConversion  OutDataTypeStr=uint16  ConvertRealWorld=Stored Integer (SI)  RndMeth=Simplest
  If : If
  If Action Subsystem : Subsystem  TreatAsAtomicUnit=on
  If Action Subsystem1 : Subsystem  TreatAsAtomicUnit=on
  Merge : Merge
  convert_pu : Gain  Gain=1/(dlgSett.UpperSatLimit)  RndMeth=Simplest  OutDataTypeStr=Inherit: Same as input
  Out1 : Outport
  wires:
  In1/1 -> convert_pu/1
  If/1 -> If Action Subsystem/Action
  If/2 -> If Action Subsystem1/Action
  convert_pu/1 -> Compare To Zero/1, If Action Subsystem/1(In1), If Action Subsystem1/1(In1)
  If Action Subsystem/1(Out1) -> Merge/1
  If Action Subsystem1/1(Out1) -> Merge/2
  Compare To Zero/1 -> Data Type Conversion/1
  Data Type Conversion/1 -> If/1
  Merge/1 -> Out1/1

== system MotorControlLibSim/Start up/Logic after motor is stoped/Enabled Subsystem ==
  In1 : Inport
  Enable : EnablePort
  Detect Change : simulink/Logic and Bit Operations/Detect Change  vinit=0  OutDataTypeStr=boolean
  Out1 : Outport
  wires:
  Detect Change/1 -> Out1/1
  In1/1 -> Detect Change/1

== system MotorControlLibSim/Start up/Logic after motor is stoped/Enabled Subsystem1 ==
  Enable : EnablePort
  Add : Sum  OutDataTypeStr=uint16
  Constant : Constant  OutDataTypeStr=uint8
  Constant1 : Constant  Value=10000  OutDataTypeStr=uint16
  Relational Operator : RelationalOperator  Operator=<=  OutDataTypeStr=boolean  RndMeth=Simplest
  Unit Delay1 : UnitDelay  SampleTime=-1  HasFrameUpgradeWarning=on
  Output : Outport
  wires:
  Add/1 -> Unit Delay1/1
  Unit Delay1/1 -> Relational Operator/1, Add/1
  Constant/1 -> Add/2
  Constant1/1 -> Relational Operator/2
  Relational Operator/1 -> Output/1

== system MotorControlLibSim/CosSin/Sine-Cosine Lookup/WrapUp/If Action Subsystem ==
  In1 : Inport
  Action Port : ActionPort  ActionPortLabel=if(u1 > 0)
  Convert_back : DataTypeConversion  RndMeth=Simplest
  Convert_uint16 : DataTypeConversion  OutDataTypeStr=int16
  Data Type Duplicate : DataTypeDuplicate
  Sum : Sum  Inputs=|+-  RndMeth=Simplest  OutDataTypeStr=Inherit: Same as first input
  Out1 : Outport
  wires:
  In1/1 -> Convert_uint16/1, Sum/1, Data Type Duplicate/1
  Convert_back/1 -> Data Type Duplicate/2, Sum/2
  Sum/1 -> Out1/1
  Convert_uint16/1 -> Convert_back/1

== system MotorControlLibSim/CosSin/Sine-Cosine Lookup/WrapUp/If Action Subsystem1 ==
  In1 : Inport
  Action Port : ActionPort  ActionPortLabel=else
  Convert_back : DataTypeConversion  RndMeth=Simplest
  Convert_uint16 : DataTypeConversion  OutDataTypeStr=int16  RndMeth=Simplest
  Data Type Duplicate : DataTypeDuplicate
  Sum : Sum  Inputs=|+-  RndMeth=Simplest  OutDataTypeStr=Inherit: Same as first input
  Out1 : Outport
  wires:
  Convert_uint16/1 -> Convert_back/1
  Convert_back/1 -> Data Type Duplicate/2, Sum/2
  In1/1 -> Convert_uint16/1, Sum/1, Data Type Duplicate/1
  Sum/1 -> Out1/1
